simulink model "LinModelSimulink"  (R2020a)
settings: Solver=VariableStepAuto  StartTime=0.0  StopTime=100  RelTol=1e-3
values from neighbouring files (symbols this model uses):
  longStraight = 1006    [plotTrack.m]
  shortStraight = 201    [plotTrack.m]
  turn = 402    [plotTrack.m]
undefined symbols (not defined in the file or in its folder): a, Area, b, banking_indy, curveCenters, Cx, g, IT, KF, KR, mT, rho_0, sigbuilder_block
libraries: simulink x2
settings Model: Creator=cvalo  LastModifiedBy=cvalo

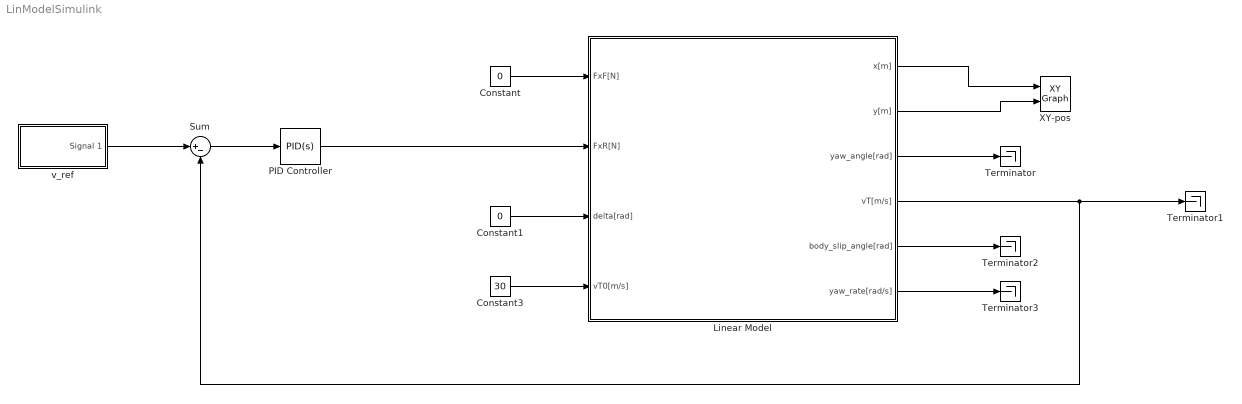
== system LinModelSimulink ==
  Constant : Constant  Value=0
  Constant1 : Constant  Value=0
  Constant3 : Constant  Value=30
  Linear Model : Subsystem
  PID Controller : simulink/Continuous/PID Controller  Controller=PID  Form=Parallel  TimeDomain=Continuous-time  UseExternalTs=off  SampleTime=-1  IntegratorMethod=Forward Euler  FilterMethod=Forward Euler  ControllerParametersSource=internal  P=1  I=1  D=0  UseFilter=on  N=100  TunerSelectOption=Transfer Function Based (PID Tuner App)  InitialConditionSource=internal  InitialConditionForIntegrator=0  InitialConditionForFilter=0  DifferentiatorICPrevScaledInput=0  ExternalReset=none  TrackingMode=off  Kt=1  LimitOutput=off  UpperSaturationLimit=inf  LowerSaturationLimit=-inf  LinearizeAsGain=on  AntiWindupMode=none  Kb=1  POutMin=[]  POutMax=[]  IOutMin=[]  IOutMax=[]  DOutMin=[]  DOutMax=[]  NOutMin=[]  NOutMax=[]  SumOutMin=[]  SumOutMax=[]  SaturationOutMin=[]  SaturationOutMax=[]  PParamMin=[]  PParamMax=[]  IParamMin=[]  IParamMax=[]  DParamMin=[]  DParamMax=[]  NParamMin=[]  NParamMax=[]  KbParamMin=[]  KbParamMax=[]  KtParamMin=[]  KtParamMax=[]  KbOutMin=[]  KbOutMax=[]  KtOutMin=[]  KtOutMax=[]  IntegratorOutMin=[]  IntegratorOutMax=[]  FilterOutMin=[]  FilterOutMax=[]  SumI1OutMin=[]  SumI1OutMax=[]  SumI2OutMin=[]  SumI2OutMax=[]  SumI3OutMin=[]  SumI3OutMax=[]  SumI4OutMin=[]  SumI4OutMax=[]  SumDOutMin=[]  SumDOutMax=[]  DifferentiatorOutMin=[]  DifferentiatorOutMax=[]  FilterDiffOutCoefMin=[]  FilterDiffOutCoefMax=[]  ReciprocalOutMin=[]  ReciprocalOutMax=[]  SumDenOutMin=[]  SumDenOutMax=[]  SumNumOutMin=[]  SumNumOutMax=[]  DivideOutMin=[]  DivideOutMax=[]  UdiffTsProdOutMin=[]  UdiffTsProdOutMax=[]  NTsProdOutMin=[]  NTsProdOutMax=[]  UintegralTsProdOutMin=[]  UintegralTsProdOutMax=[]  UngainTsProdOutMin=[]  UngainTsProdOutMax=[]  IntegratorContinuousStateAttributes=''  IntegratorStateMustResolveToSignalObject=off  IntegratorRTWStateStorageClass=Auto  FilterContinuousStateAttributes=''  FilterStateMustResolveToSignalObject=off  FilterRTWStateStorageClass=Auto  ParallelPVariant=InternalParameters  IdealPVariant=Disabled  IVariant=InternalParameters  DVariant=InternalParameters  IntegratorVariant=Continuous  SatVariant=Disabled  AWVariant=Passthrough  PCopyVariant=Disabled  TRVariant=Disabled  FdbkBlocksVariant=Forward  IdealPFdbkVariant=Disabled  SatFdbkVariant=Disabled  DerivativeFilterVariant=ContFilter  NVariant=InternalParameters  NCopyVariant=Disabled  FilterICVariant=InternalICsFilter  IntegratorICVariant=InternalICs  ExternalResetVariant=Disabled  TRSumVariant=Passthrough  SumFdbkVariant=Disabled  SumVariant=Sum_PID  TsampFilterVariant=InternalTs  TsampNgainVariant=Passthrough  TsampIntegralVariant=Passthrough
  Sum : Sum  Inputs=|+-
  Terminator{,1..3} (4 alike) : Terminator
  XY-pos : simulink/Sinks/XY Graph  xmin=-10  xmax=3100  ymin=-10  ymax=20  st=-1
  v_ref : Subsystem  Tag=STV Subsys  LoadFcn=sigbuilder_block('load');  StartFcn=sigbuilder_block('start');  StopFcn=sigbuilder_block('stop');  ClipboardFcn=sigbuilder_block('clipboard');  mask(Sigbuilder block){tuvar=[0:10]}
      mask help: Simulink:masks:SigbuilderBlock_MD
      mask init:
      | if ~strcmp(get_param(bdroot(gcbh),'SimulationStatus'),'stopped') tuvar = sigbuilder_block('maskInit'); end
      settings: CopyFcn=sigbuilder_block('copy');  DeleteFcn=sigbuilder_block('delete');  ModelCloseFcn=sigbuilder_block('modelClose');  PreSaveFcn=sigbuilder_block('preSave');  PauseFcn=sigbuilder_block('pause');  ContinueFcn=sigbuilder_block('continue');  NameChangeFcn=sigbuilder_block('namechange');  OpenFcn=sigbuilder_block('open',[0 30 1152 561.6 ]);  CloseFcn=sigbuilder_block('close');
      mask Display: plot(0, 0, 100, 100,[2, 2, 32, 32, 2], [68, 8, 8, 68, 68],[32, 2], [38, 38], [32, 19, 2],[53, 60, 44], [32, 17, 17, 2],[16, 16, 31, 31]);txt = getActiveGroup(gcbh);text(2, 100, txt,'verticalAlignment', 'top');
  wires:
  Linear Model/1(x[m]) -> XY-pos/1
  Linear Model/2(y[m]) -> XY-pos/2
  Linear Model/3(yaw_angle[rad]) -> Terminator/1
  Linear Model/4(vT[m/s]) -> Sum/2, Terminator1/1
  Linear Model/5(body_slip_angle[rad]) -> Terminator2/1
  Linear Model/6(yaw_rate[rad/s]) -> Terminator3/1
  Constant/1 -> Linear Model/1(FxF[N])
  Constant1/1 -> Linear Model/3(delta[rad])
  PID Controller/1 -> Linear Model/2(FxR[N])
  Constant3/1 -> Linear Model/4(vT0[m/s])
  Sum/1 -> PID Controller/1
  v_ref/1(Signal 1) -> Sum/1

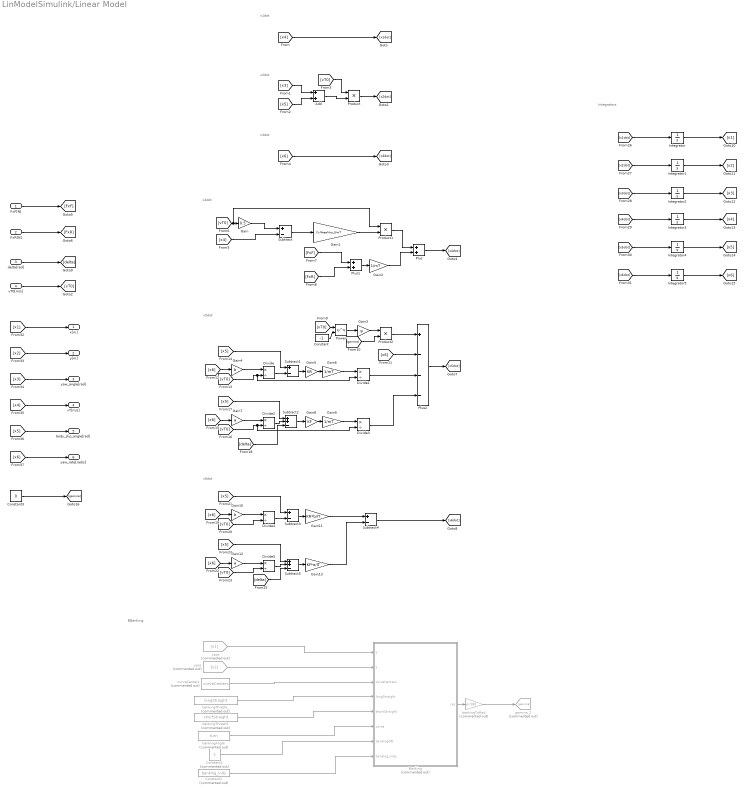
== system LinModelSimulink/Linear Model ==
  note: BBanking
  note: Integrators
  note: x1dot
  note: x2dot
  note: x3dot
  note: x4dot
  note: x5dot
  note: x6dot
  FxF[N] : Inport  Unit=N
  FxR[N] : Inport  Port=2  Unit=N
  delta[rad] : Inport  Port=3  Unit=N
  vT0[m/s] : Inport  Port=4  Unit=m/s
  Add : Sum
  Banking : MATLAB Function  Commented=on  TreatAsAtomicUnit=on
  Constant : Constant  Value=-1
  Constant1 : Constant  Commented=on  Value=banking_indy
  Constant2 : Constant  Commented=on
  Constant3 : Constant  Value=0
  Divide{,1..5} (6 alike) : Product  Inputs=*/
  Gain : Gain  Gain=0.5
  Gain1 : Gain  Gain=Cx*Area*rho_0/mT
  Gain10 : Gain  Gain=b
  Gain11 : Gain  Gain=KR*b/IT
  Gain12 : Gain  Gain=a
  Gain13 : Gain  Gain=KF*a/IT
  Gain2 : Gain  Gain=1/mT
  Gain3 : Gain  Gain=g
  Gain4 : Gain  Gain=b
  Gain5 : Gain  Gain=KR
  Gain6 : Gain  Gain=1/mT
  Gain7 : Gain  Gain=a
  Gain8 : Gain  Gain=KF
  Gain9 : Gain  Gain=1/mT
  Integrator{,1..2,4..5} (5 alike) : Integrator
  Integrator3 : Integrator  InitialCondition=25  LimitOutput=on  LowerSaturationLimit=0
  Plus : Sum
  Plus1 : Sum
  Plus2 : Sum  Inputs=+---
  Power : Math  Operator=pow  SaturateOnIntegerOverflow=on
  Product : Product
  Product1 : Product
  Product2 : Product
  Subtract{,1,3..4} (4 alike) : Sum  Inputs=+-
  Subtract2 : Sum  Inputs=++-
  Subtract5 : Sum  Inputs=++-
  bankingAngle : Constant  Commented=on  Value=turn
  bankingThreshL : Constant  Commented=on  Value=longStraight
  bankingThreshS : Constant  Commented=on  Value=shortStraight
  bankingToRad : Gain  Commented=on  Gain=pi/180
  curveCenters : Constant  Commented=on  Value=curveCenters
  gamma_2 : Goto  Commented=on  GotoTag=gamma
  xpos : From  Commented=on  GotoTag=x1
  ypos : From  Commented=on  GotoTag=x2
  x[m] : Outport  Unit=m
  y[m] : Outport  Port=2  Unit=m
  yaw_angle[rad] : Outport  Port=3  Unit=rad
  vT[m/s] : Outport  Port=4  Unit=m/s
  body_slip_angle[rad] : Outport  Port=5  Unit=rad
  yaw_rate[rad/s] : Outport  Port=6  Unit=rad/s
  wires:
  Integrator4/1 -> [x5]
  [x6] -> [x3dot]
  [x2] -> y[m]/1
  [x3] -> yaw_angle[rad]/1
  [x6] -> yaw_rate[rad/s]/1
  [vT0] -> Divide1/2, Divide/2
  Integrator5/1 -> [x6]
  [x1] -> x[m]/1
  [x4dot] -> Integrator3/1
  [x5] -> Subtract5/1
  Gain/1 -> Subtract/1
  [x4] -> [x1dot]
  [x5dot] -> Integrator4/1
  Gain5/1 -> Gain6/1
  Integrator1/1 -> [x2]
  Gain10/1 -> Divide4/1
  Gain2/1 -> Plus/2
  Divide3/1 -> Plus2/4
  [vT0] -> Product1/1, Gain/1
  bankingToRad/1 -> gamma_2/1
  Product/1 -> [x2dot]
  Divide1/1 -> Plus2/3
  [x6] -> Gain4/1
  Constant1/1 -> Banking/8(banking_indy)
  [FxR] -> Plus1/2
  Power/1 -> Gain3/1
  Plus1/1 -> Gain2/1
  Gain11/1 -> Subtract4/1
  [x3] -> Add/1
  [x5] -> Subtract3/1
  [x5] -> Add/2
  [x4] -> Subtract/2
  [gamma] -> Product2/2
  [vT0] -> Divide4/2
  vT0[m/s]/1 -> [vT0]
  Add/1 -> Product/2
  FxF[N]/1 -> [FxF]
  ypos/1 -> Banking/2(y)
  delta[rad]/1 -> [delta]
  [FxF] -> Plus1/1
  [vT0] -> Product/1
  Gain1/1 -> Product1/2
  bankingAngle/1 -> Banking/6(curve)
  Plus/1 -> [x4dot]
  Product1/1 -> Plus/1
  [x2dot] -> Integrator1/1
  [x6] -> Gain10/1
  [x6] -> Plus2/2
  Subtract/1 -> Gain1/1
  [x4] -> vT[m/s]/1
  FxR[N]/1 -> [FxR]
  [x5] -> Subtract1/1
  Banking/1(res) -> bankingToRad/1
  Constant/1 -> Power/2
  Gain4/1 -> Divide/1
  [vT0] -> Power/1
  Plus2/1 -> [x5dot]
  curveCenters/1 -> Banking/3(curveCenters)
  Divide/1 -> Subtract1/2
  Gain3/1 -> Product2/1
  bankingThreshL/1 -> Banking/4(longStraight)
  bankingThreshS/1 -> Banking/5(shortStraight)
  xpos/1 -> Banking/1(x)
  [x1dot] -> Integrator/1
  Product2/1 -> Plus2/1
  [x6dot] -> Integrator5/1
  Integrator/1 -> [x1]
  Integrator3/1 -> [x4]
  Subtract4/1 -> [x6dot]
  [delta] -> Subtract5/3
  Subtract5/1 -> Gain13/1
  [x6] -> Gain12/1
  Divide5/1 -> Subtract5/2
  [vT0] -> Divide5/2
  Gain12/1 -> Divide5/1
  Subtract1/1 -> Gain5/1
  Gain13/1 -> Subtract4/2
  Subtract3/1 -> Gain11/1
  [delta] -> Subtract2/3
  [vT0] -> Divide3/2, Divide2/2
  Gain8/1 -> Gain9/1
  Gain9/1 -> Divide3/1
  [x5] -> Subtract2/1
  Subtract2/1 -> Gain8/1
  Divide2/1 -> Subtract2/2
  [x6] -> Gain7/1
  Gain6/1 -> Divide1/1
  Gain7/1 -> Divide2/1
  [x3dot] -> Integrator2/1
  Integrator2/1 -> [x3]
  Divide4/1 -> Subtract3/2
  [x5] -> body_slip_angle[rad]/1
  Constant2/1 -> Banking/7(bankingON)
  Constant3/1 -> [gamma]

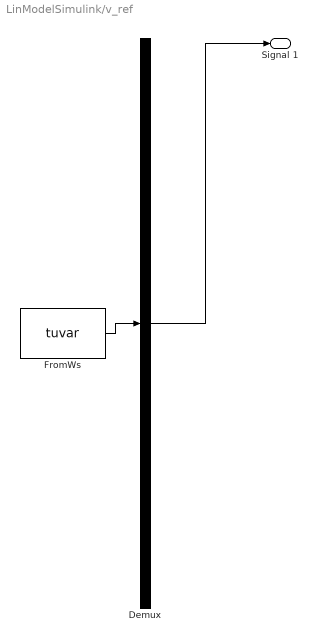
== system LinModelSimulink/v_ref ==
  Demux : Demux  Tag=STV Demux  Outputs=1
      settings: DisplayOption=none
  FromWs : FromWorkspace  Tag=STV FromWs  VariableName=tuvar
      SigBuilderData=|
      | common.afterFinalStr = 'Extrapolate'
      | common.sampleTime = 0
      | dataSet.timeRange = [0 100]
      | dataSet.name = 'Group 1'
      | sbobj.Groups.Name = 'Group 1'
      | sbobj.Groups.Signals.Name = 'Signal 1'
      | sbobj.Groups.Signals.XData = [0 4.2 6.3 20.7 28.3 42.3 49.7 67.5 100]
      | sbobj.Groups.Signals.YData = [30.4275 30.4275 31.3 41.45 38.95 36.35 31.9 35.15 35.2]
      | sbobj.Groups.TimeRange = [0 100]
  Signal 1 : Outport  Tag=STV Outport
  wires:
  Demux/1 -> Signal 1/1
  FromWs/1 -> Demux/1

== matlab function LinModelSimulink/Linear Model/Banking ==
  data: x input; res output; y input; curveCenters input; longStraight input; shortStraight input; curve input; bankingON input; banking_indy input
function res = calculateBanking(x, y, curveCenters, ...
    longStraight, shortStraight, curve, ...
    bankingON, banking_indy)

% coder.extrinsic('evalin')
% coder.extrinsic('fitresult')
% fun = evalin('base','fitresult');

init_x = -271.4;
totL = 4023.4;
initD = pdist2([init_x, 0], [curveCenters(1,1),0]);

R = curve * 2 / pi;


if (bankingON < 1)
    res = 0;
else
    % long straight 1
    if y < curveCenters(1,2) && x >= curveCenters(4,1) && x <= curveCenters(1,1)
        d = pdist2([x, 0],[init_x, 0]);
        l = (totL - d)*(x < init_x) + ...
            (d)*(x >= init_x);
    % long straight 2
    elseif y > curveCenters(2,2) && x >= curveCenters(4,1) && x <= curveCenters(1,1)
        d = pdist2([x, 0],[curveCenters(2,1),0]);
        l = d + initD + shortStraight + 2*curve;
    % short straigt 1
    elseif x > 0 && y >= curveCenters(1,2) && y <= curveCenters(2,2)
        d = pdist2([y, 0],[curveCenters(1,2),0]);
        l = d + initD + curve;
    % short straigt 2
    elseif x < 0 && y >= curveCenters(1,2) && y <= curveCenters(2,2)
        d = pdist2([y, 0],[curveCenters(3,2),0]);
        l = d + initD + longStraight + shortStraight + 3*curve;
    % curve 1
    elseif x > curveCenters(1,1) && y < curveCenters(1,2)
        ang = asin((x - curveCenters(1,1))/pdist2([x,y],curveCenters(1,:)));
        l = ang * R + initD;
    % curve 2
    elseif x > curveCenters(2,1) && y > curveCenters(2,2)
        ang = asin((y - curveCenters(2,2))/pdist2([x,y],curveCenters(2,:)));
        l = ang * R + initD + curve + shortStraight;
    % curve 3
    elseif x < curveCenters(3,1) && y > curveCenters(3,2)
        ang = asin((-x + curveCenters(3,1))/pdist2([x,y],curveCenters(3,:)));
        l = ang * R + initD + curve*2 + shortStraight + longStraight;
    % curve 4
    elseif x < curveCenters(4,1) && y < curveCenters(4,2)
        ang = asin((-y + curveCenters(4,2))/pdist2([x,y],curveCenters(4,:)));
        l = ang * R + initD + curve*3 + shortStraight*2 + longStraight;
    % default else
    else 
        l = 0;
    end
    
    %res = fun(l);
    res = banking_indy(ceil(l*10),1);
    %res = 0;
end

% function res = calculateBanking(x, y, curveCenters, ...
%     bankingThresholdLong, bankingThresholdShort, bankingAngle, midY, ...
%     bankingON)
% if (bankingON < 1)
%     res = 0;
% else
%     if(y < curveCenters(1,2) || y > curveCenters(2,2)) 
%        if(abs(x) < curveCenters(1,1) - bankingThresholdLong)
%            res = 0;
%        elseif (abs(x) > curveCenters(1,1))
%            res = bankingAngle;
%        else
%            res = bankingAngle*( 1 - ((abs(x) -  curveCenters(1,1))/(-bankingThresholdLong)) );
%        end
%     else
%         if (abs(y-midY) < curveCenters(2,2) - bankingThresholdShort - midY)
%             res = 0;
%         else
%             res = bankingAngle*( 1 - ((abs(y-midY) -  curveCenters(2,2) + midY)/(-bankingThresholdShort)) );
%         end
%     end
% end
